simulink model "track"  (R2019a)
settings: Solver=VariableStepAuto  StartTime=0.0  StopTime=10.0  RelTol=1e-3
settings Model: Creator=张涛  LastModifiedBy=张涛
settings DataIOCC: SaveFormat=Array  ReturnWorkspaceOutputs=off

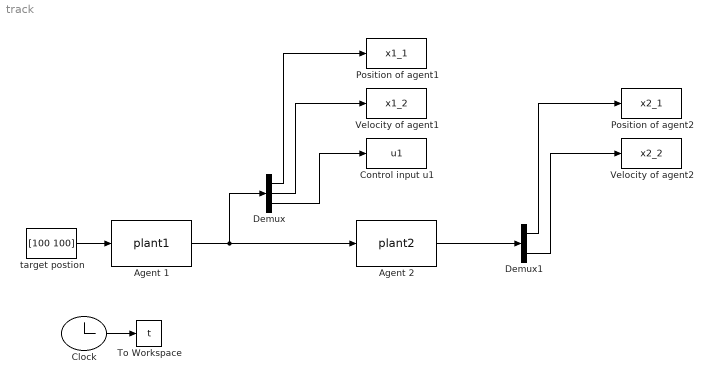
== system track ==
  Agent 1 : S-Function  FunctionName=plant1  Parameters=[0 0 0 0]  SFunctionDeploymentMode=off  EnableBusSupport=off
  Agent 2 : S-Function  FunctionName=plant2  Parameters=[60 5 0 0]  SFunctionDeploymentMode=off  EnableBusSupport=off
  Clock : Clock
  Control input u1 : ToWorkspace  VariableName=u1  SampleTime=-1
  Demux : Demux  Outputs=3
  Demux1 : Demux  Outputs=2
  Position of agent1 : ToWorkspace  VariableName=x1_1  SampleTime=-1
  Position of agent2 : ToWorkspace  VariableName=x2_1  SampleTime=-1
  To Workspace : ToWorkspace  VariableName=t  SampleTime=-1
  Velocity of agent1 : ToWorkspace  VariableName=x1_2  SampleTime=-1
  Velocity of agent2 : ToWorkspace  VariableName=x2_2  SampleTime=-1
  target postion : Constant  Value=[100 100]
  wires:
  Agent 1/1 -> Demux/1, Agent 2/1
  target postion/1 -> Agent 1/1
  Clock/1 -> To Workspace/1
  Demux/1 -> Position of agent1/1
  Demux/2 -> Velocity of agent1/1
  Demux/3 -> Control input u1/1
  Demux1/1 -> Position of agent2/1
  Demux1/2 -> Velocity of agent2/1
  Agent 2/1 -> Demux1/1
